simulink library "BdotController"  (R2018a)
settings: Solver=ode45  StartTime=0.0  StopTime=10.0  RelTol=1e-3  EnableMultiTasking=on
undefined symbols (not defined in the file): ConfParam
libraries: RWS_1W_PDcontroller x2, ComputeNorm3D x1
settings Model: Creator=Hp  LastModifiedBy=Cédric
settings DataIOCC: LimitDataPoints=on  SaveFormat=Array
settings OptimizationCC: LifeSpan=inf
settings DebuggingCC: SolverPrmCheckMsg=warning  SFUnexpectedBacktrackingDiag=warning  SFNoUnconditionalDefaultTransitionDiag=warning  SFExecutionAtInitializationDiag=none
settings HardwareCC: ProdBitPerPointer=32  ProdBitPerSizeT=32  ProdBitPerPtrDiffT=32  ProdLargestAtomicFloat=None  ProdIntDivRoundTo=Undefined  ProdEndianess=Unspecified  ProdWordSize=32  ProdHWDeviceType=32-bit Generic
settings ModelReferenceCC: PropagateSignalLabelsOutOfModel=off
settings CodeAppCC: StateflowObjectComments=on
settings GRTTargetCC: TargetLangStandard=C89/C90 (ANSI)  GeneratePreprocessorConditionals=Disable all
settings ConfigComp: CovMetricSettings=dw  CovHtmlReporting=on  CovSaveCumulativeToWorkspaceVar=on  CovSaveSingleToWorkspaceVar=on  CovExternalEMLEnable=off  CovSFcnEnable=off

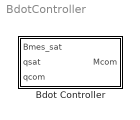
== system BdotController ==
  Bdot Controller : Subsystem

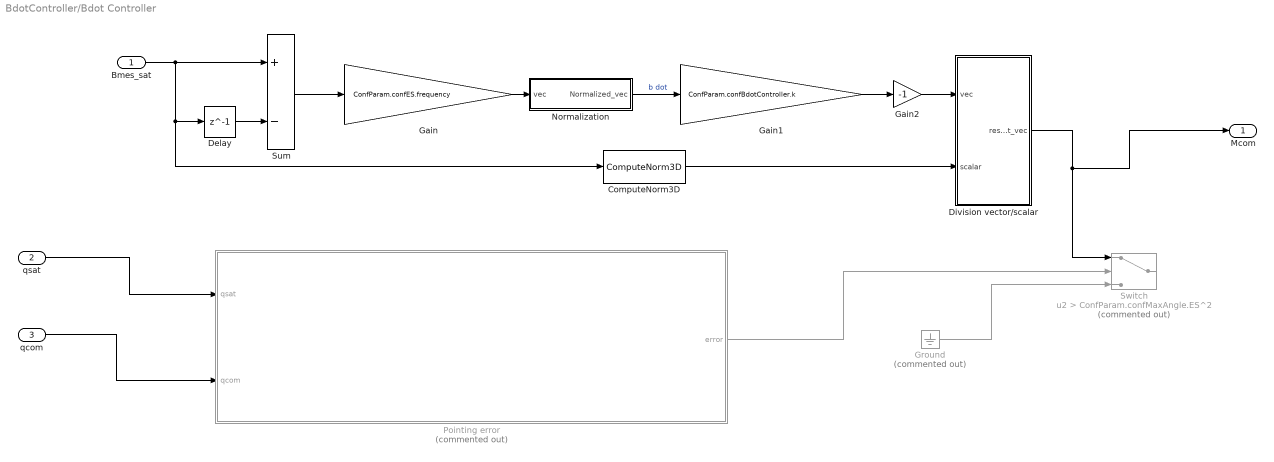
== system BdotController/Bdot Controller ==
  Bmes_sat : Inport
  qsat : Inport  Port=2
  qcom : Inport  Port=3
  ComputeNorm3D : ComputeNorm3D/ComputeNorm3D
  Delay : Delay  DelayLength=1  InitialCondition=[0;0;0]  SampleTime=1/ConfParam.confES.frequency
  Division vector/scalar : Subsystem
  Gain : Gain  Gain=ConfParam.confES.frequency
  Gain1 : Gain  Gain=ConfParam.confBdotController.k
  Gain2 : Gain  Gain=-1
  Ground : Ground  Commented=on
  Normalization : Subsystem
  Pointing error : Subsystem  Commented=on
  Sum : Sum  Inputs=+-
  Switch : Switch  Commented=on  Criteria=u2 > Threshold  Threshold=ConfParam.confMaxAngle.ES^2
  Mcom : Outport
  wires:
  Sum/1 -> Gain/1
  Normalization/1(Normalized_vec) -> Gain1/1  "b dot"
  Gain1/1 -> Gain2/1
  Gain2/1 -> Division vector/scalar/1(vec)
  ComputeNorm3D/1 -> Division vector/scalar/2(scalar)
  Gain/1 -> Normalization/1(vec)
  Bmes_sat/1 -> ComputeNorm3D/1, Delay/1, Sum/1
  Delay/1 -> Sum/2
  Ground/1 -> Switch/3
  Division vector/scalar/1(result_vec) -> Mcom/1, Switch/1
  qsat/1 -> Pointing error/1(qsat)
  qcom/1 -> Pointing error/2(qcom)
  Pointing error/1(error) -> Switch/2

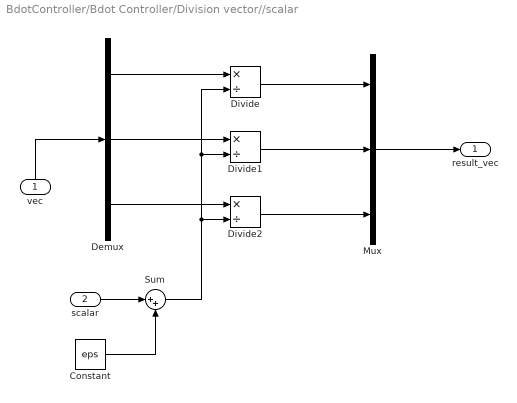
== system BdotController/Bdot Controller/Division vector//scalar ==
  vec : Inport
  scalar : Inport  Port=2
  Constant : Constant  Value=eps  SampleTime=1/ConfParam.confES.frequency
  Demux : Demux  Outputs=3
  Divide : Product  Inputs=*/
  Divide1 : Product  Inputs=*/
  Divide2 : Product  Inputs=*/
  Mux : Mux  Inputs=3
  Sum : Sum  Inputs=|++
  result_vec : Outport
  wires:
  scalar/1 -> Sum/1
  Constant/1 -> Sum/2
  Divide/1 -> Mux/1
  Mux/1 -> result_vec/1
  Sum/1 -> Divide1/2, Divide/2, Divide2/2
  Demux/3 -> Divide2/1
  Divide2/1 -> Mux/3
  Divide1/1 -> Mux/2
  Demux/1 -> Divide/1
  Demux/2 -> Divide1/1
  vec/1 -> Demux/1

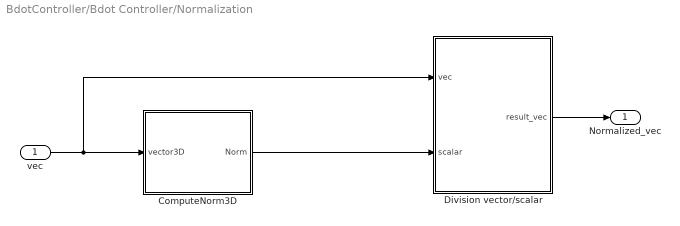
== system BdotController/Bdot Controller/Normalization ==
  vec : Inport
  ComputeNorm3D : Subsystem
  Division vector/scalar : Subsystem
  Normalized_vec : Outport
  wires:
  ComputeNorm3D/1(Norm) -> Division vector/scalar/2(scalar)
  Division vector/scalar/1(result_vec) -> Normalized_vec/1
  vec/1 -> ComputeNorm3D/1(vector3D), Division vector/scalar/1(vec)

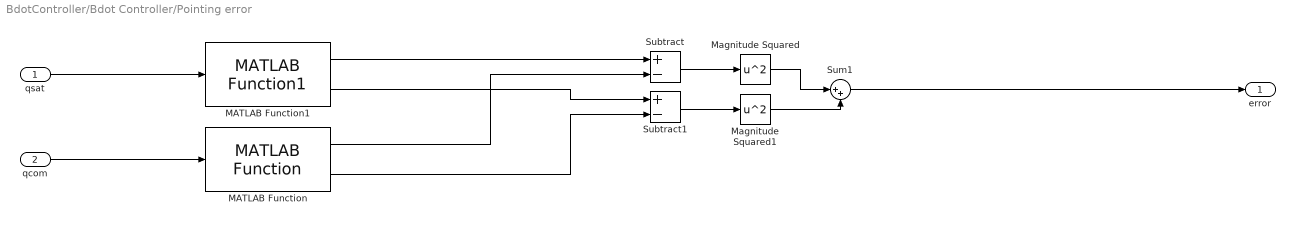
== system BdotController/Bdot Controller/Pointing error ==
  qsat : Inport
  qcom : Inport  Port=2
  MATLAB Function : RWS_1W_PDcontroller/RWS 1W PD controller/Bang-bang control law/MATLAB Function
  MATLAB Function1 : RWS_1W_PDcontroller/RWS 1W PD controller/Bang-bang control law/MATLAB Function1
  Magnitude Squared : Math  Operator=square  SaturateOnIntegerOverflow=on
  Magnitude Squared1 : Math  Operator=square  SaturateOnIntegerOverflow=on
  Subtract : Sum  Inputs=+-
  Subtract1 : Sum  Inputs=+-
  Sum1 : Sum  Inputs=|++
  error : Outport
  wires:
  MATLAB Function/2 -> Subtract1/2
  Sum1/1 -> error/1
  MATLAB Function1/1 -> Subtract/1
  Magnitude Squared1/1 -> Sum1/2
  Magnitude Squared/1 -> Sum1/1
  Subtract/1 -> Magnitude Squared/1
  MATLAB Function/1 -> Subtract/2
  Subtract1/1 -> Magnitude Squared1/1
  MATLAB Function1/2 -> Subtract1/1
  qsat/1 -> MATLAB Function1/1
  qcom/1 -> MATLAB Function/1

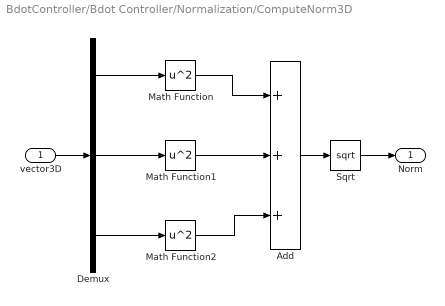
== system BdotController/Bdot Controller/Normalization/ComputeNorm3D ==
  vector3D : Inport
  Add : Sum  Inputs=+++
  Demux : Demux  Outputs=3
  Math Function : Math  Operator=square  SaturateOnIntegerOverflow=on
  Math Function1 : Math  Operator=square  SaturateOnIntegerOverflow=on
  Math Function2 : Math  Operator=square  SaturateOnIntegerOverflow=on
  Sqrt : Sqrt  SaturateOnIntegerOverflow=on
  Norm : Outport
  wires:
  Demux/2 -> Math Function1/1
  Demux/3 -> Math Function2/1
  Math Function/1 -> Add/1
  Demux/1 -> Math Function/1
  Math Function2/1 -> Add/3
  Math Function1/1 -> Add/2
  Add/1 -> Sqrt/1
  Sqrt/1 -> Norm/1
  vector3D/1 -> Demux/1

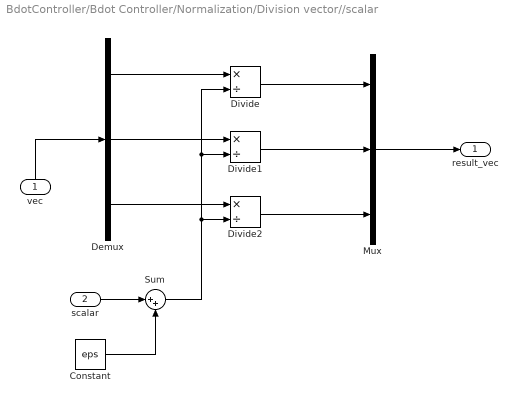
== system BdotController/Bdot Controller/Normalization/Division vector//scalar ==
  vec : Inport
  scalar : Inport  Port=2
  Constant : Constant  Value=eps  SampleTime=1/ConfParam.confES.frequency
  Demux : Demux  Outputs=3
  Divide : Product  Inputs=*/
  Divide1 : Product  Inputs=*/
  Divide2 : Product  Inputs=*/
  Mux : Mux  Inputs=3
  Sum : Sum  Inputs=|++
  result_vec : Outport
  wires:
  scalar/1 -> Sum/1
  Constant/1 -> Sum/2
  Divide/1 -> Mux/1
  Mux/1 -> result_vec/1
  Sum/1 -> Divide1/2, Divide/2, Divide2/2
  Demux/3 -> Divide2/1
  Divide2/1 -> Mux/3
  Divide1/1 -> Mux/2
  Demux/1 -> Divide/1
  Demux/2 -> Divide1/1
  vec/1 -> Demux/1
